simulink model "Stan_Ilya_314_4_2"  (R2018a)
settings: Solver=VariableStepAuto  StartTime=0.0  StopTime=100  RelTol=1e-3
libraries: simulink x1
settings Model: Creator=ilya  LastModifiedBy=ilya

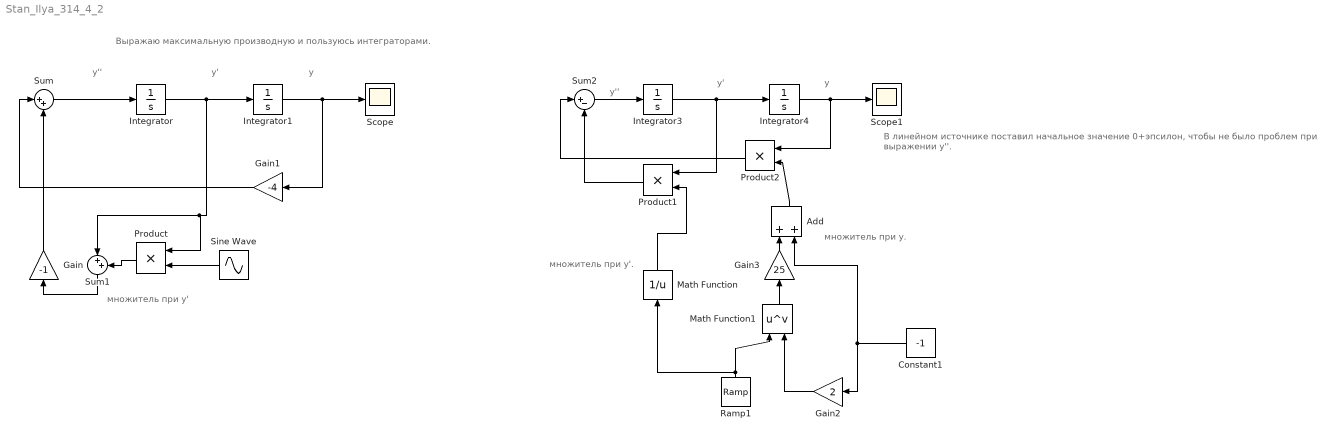
== system Stan_Ilya_314_4_2 ==
  note: Выражаю максимальную производную и пользуюсь интеграторами.
  note: множитель при y'
  note: множитель при у'.
  note: множитель при y.
  note: В линейном источнике поставил начальное значение 0+эпсилон, чтобы не было проблем при выражении у''.
  note: y''
  note: y
  note: y'
  note: y
  note: y'
  note: y''
  Add : Sum
  Constant1 : Constant  Value=-1
  Gain : Gain  Gain=-1
  Gain1 : Gain  Gain=-4
  Gain2 : Gain  Gain=2
  Gain3 : Gain  Gain=25
  Integrator : Integrator  InitialCondition=1
  Integrator1 : Integrator  InitialCondition=2
  Integrator3 : Integrator  InitialCondition=10
  Integrator4 : Integrator  InitialCondition=1
  Math Function : Math  Operator=reciprocal  SaturateOnIntegerOverflow=on
  Math Function1 : Math  Operator=pow  SaturateOnIntegerOverflow=on
  Product : Product
  Product1 : Product
  Product2 : Product
  Ramp1 : simulink/Sources/Ramp  slope=1  start=0  InitialOutput=0.0001
  Scope : Scope
  Scope1 : Scope
  Sine Wave : Sin  Amplitude=-0.5  Phase=pi/2  SampleTime=0
  Sum : Sum  Inputs=|++
  Sum1 : Sum  Inputs=|++
  Sum2 : Sum  Inputs=|+-
  wires:
  Integrator1/1 -> Scope/1, Gain1/1
  Sum/1 -> Integrator/1
  Gain1/1 -> Sum/1
  Integrator/1 -> Product/1, Sum1/1, Integrator1/1
  Sum1/1 -> Gain/1
  Gain/1 -> Sum/2
  Product/1 -> Sum1/2
  Sine Wave/1 -> Product/2
  Integrator3/1 -> Product1/1, Integrator4/1
  Integrator4/1 -> Product2/1, Scope1/1
  Ramp1/1 -> Math Function1/1, Math Function/1
  Sum2/1 -> Integrator3/1
  Gain2/1 -> Math Function1/2
  Math Function/1 -> Product1/2
  Product1/1 -> Sum2/2
  Math Function1/1 -> Gain3/1
  Constant1/1 -> Add/2, Gain2/1
  Add/1 -> Product2/2
  Product2/1 -> Sum2/1
  Gain3/1 -> Add/1
